simulink model "Test_Adder"  (Simulink 8.1)
settings: Solver=ode45  StartTime=0.0  StopTime=10.0  RelTol=1e-3
libraries: Computer_Library x2
settings Model: Creator=N  LastModifiedBy=uzivatel
settings DataIOCC: LimitDataPoints=off  SignalLoggingSaveFormat=Dataset
settings OptimizationCC: ExpressionDepthLimit=128
settings DebuggingCC: UnderspecifiedInitializationDetection=Simplified  MergeDetectMultiDrivingBlocksExec=error  SolverPrmCheckMsg=none  FcnCallInpInsideContextMsg=EnableAllAsError  FrameProcessingCompatibilityMsg=error  StateNameClashWarn=none
settings HardwareCC: ProdBitPerPointer=64  ProdLargestAtomicFloat=Float  ProdIntDivRoundTo=Zero  ProdEndianess=LittleEndian  ProdHWDeviceType=Intel->x86-64 (Windows64)
settings ModelReferenceCC: PropagateSignalLabelsOutOfModel=on
settings GRTTargetCC: CodeReplacementLibrary=None  CombineOutputUpdateFcns=on  CPPClassGenCompliant=on  GRTInterface=off

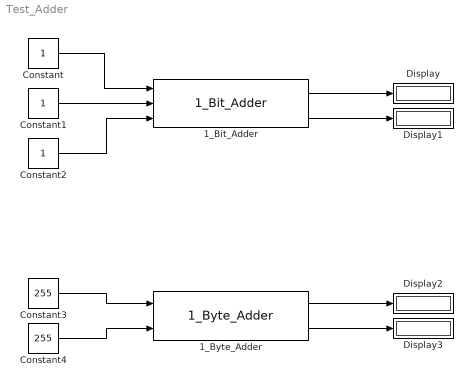
== system Test_Adder ==
  1_Bit_Adder : Computer_Library/Adders/1_Bit_Adder
  1_Byte_Adder : Computer_Library/Adders/1_Byte_Adder
  Constant : Constant
  Constant1 : Constant
  Constant2 : Constant
  Constant3 : Constant  Value=255
  Constant4 : Constant  Value=255
  Display{,1..3} (4 alike) : Display
  wires:
  1_Bit_Adder/1 -> Display/1
  1_Bit_Adder/2 -> Display1/1
  Constant/1 -> 1_Bit_Adder/1
  Constant1/1 -> 1_Bit_Adder/2
  Constant2/1 -> 1_Bit_Adder/3
  1_Byte_Adder/2 -> Display3/1
  Constant3/1 -> 1_Byte_Adder/1
  Constant4/1 -> 1_Byte_Adder/2
  1_Byte_Adder/1 -> Display2/1
